simulink model "Simulation_labo4_r2015a"  (R2015a)
settings: Solver=ode15s  StartTime=0.0  StopTime=0.3  RelTol=1e-3
undefined symbols (not defined in the file): bmg, bmm, consigne, jeq, Ka, kbm, Kd, Ki, kmm, Kp, lam, ram, temps_test
settings Model: CovModelRefEnable=off  Creator=ak71840  LastModifiedBy=Oatmeal
settings DataIOCC: SaveFormat=Dataset
settings HardwareCC: ProdBitPerPointer=64  ProdLargestAtomicFloat=Float  ProdIntDivRoundTo=Zero  ProdEndianess=LittleEndian  ProdHWDeviceType=Specified
settings GRTTargetCC: GeneratePreprocessorConditionals=Use local settings

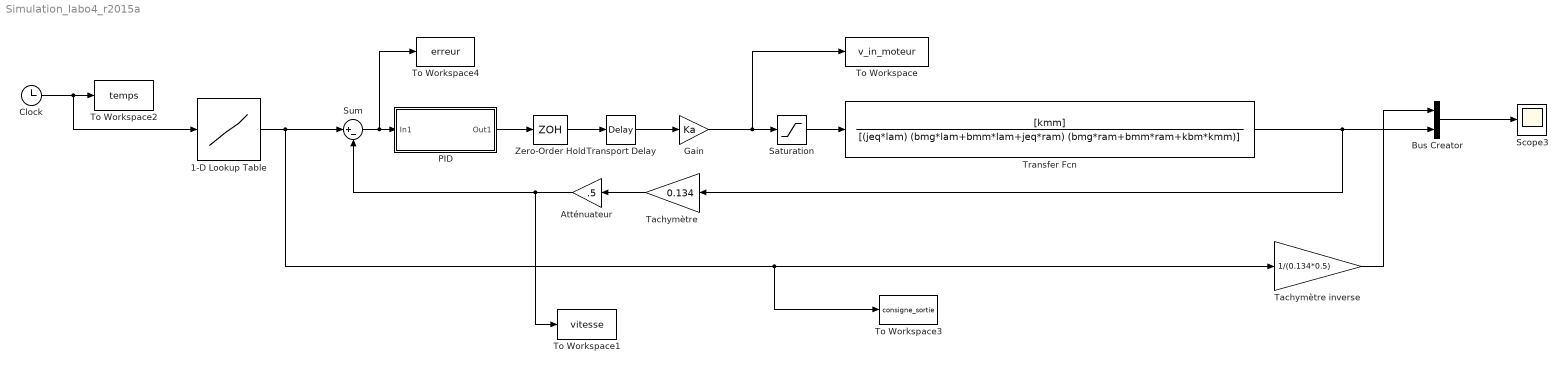
== system Simulation_labo4_r2015a ==
  1-D Lookup Table : Lookup_n-D  NumberOfTableDimensions=1  BreakpointsForDimension1=temps_test  Table=consigne  InternalRulePriority=Speed  RndMeth=Simplest  InputSameDT=on
  Atténuateur : Gain  Gain=.5
  Bus Creator : BusCreator  Inputs=2
  Clock : Clock
  Gain : Gain  Gain=Ka
  PID : Subsystem  TreatAsAtomicUnit=on
  Saturation : Saturate  UpperLimit=20  LowerLimit=-20
  Scope3 : Scope
      settings: SaveName=ScopeData3
  Sum : Sum  Inputs=|+-
  Tachymètre : Gain  Gain=0.134
  Tachymètre inverse : Gain  Gain=1/(0.134*0.5)
  To Workspace : ToWorkspace  VariableName=v_in_moteur  SampleTime=-1
  To Workspace1 : ToWorkspace  VariableName=vitesse  SampleTime=-1
  To Workspace2 : ToWorkspace  VariableName=temps  SampleTime=-1
  To Workspace3 : ToWorkspace  VariableName=consigne_sortie  SampleTime=-1
  To Workspace4 : ToWorkspace  VariableName=erreur  SampleTime=-1
  Transfer Fcn : TransferFcn  Numerator=[kmm]  Denominator=[(jeq*lam) (bmg*lam+bmm*lam+jeq*ram) (bmg*ram+bmm*ram+kbm*kmm)]
  Transport Delay : TransportDelay  DelayTime=0.002
  Zero-Order Hold : ZeroOrderHold  SampleTime=0.005
  wires:
  1-D Lookup Table/1 -> Sum/1, Tachymètre inverse/1, To Workspace3/1
  Sum/1 -> To Workspace4/1, PID/1(In1)
  Gain/1 -> To Workspace/1, Saturation/1
  Clock/1 -> 1-D Lookup Table/1, To Workspace2/1
  Transfer Fcn/1 -> Tachymètre/1, Bus Creator/2
  PID/1(Out1) -> Zero-Order Hold/1
  Zero-Order Hold/1 -> Transport Delay/1
  Transport Delay/1 -> Gain/1
  Saturation/1 -> Transfer Fcn/1
  Bus Creator/1 -> Scope3/1
  Tachymètre/1 -> Atténuateur/1
  Atténuateur/1 -> To Workspace1/1, Sum/2
  Tachymètre inverse/1 -> Bus Creator/1

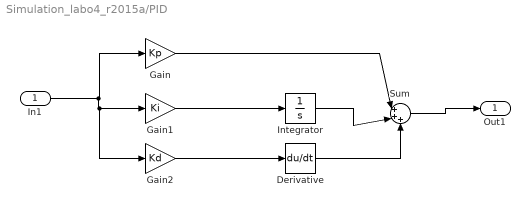
== system Simulation_labo4_r2015a/PID ==
  In1 : Inport
  Derivative : Derivative
  Gain : Gain  Gain=Kp
  Gain1 : Gain  Gain=Ki
  Gain2 : Gain  Gain=Kd
  Integrator : Integrator
  Sum : Sum  Inputs=|+++
  Out1 : Outport
  wires:
  Gain2/1 -> Derivative/1
  Gain1/1 -> Integrator/1
  Gain/1 -> Sum/1
  Integrator/1 -> Sum/2
  Derivative/1 -> Sum/3
  Sum/1 -> Out1/1
  In1/1 -> Gain/1, Gain2/1, Gain1/1
